simulink model "PID_Block"  (R2020b)
settings: Solver=VariableStepAuto  StartTime=0.0  StopTime=10.0  RelTol=1e-3
values from neighbouring files (symbols this model uses):
  Kd = 300    [mass_damper_pid.m]    (also in mass_damper_pid_improved.m = 0)
  Ki = 50    [mass_damper_pid.m]    (also in mass_damper_pid_improved.m = 0)
  Kp = 500    [mass_damper_pid.m]    (also in mass_damper_pid_improved.m)
settings Model: Creator=Raihan mahmud  LastModifiedBy=Raihan mahmud

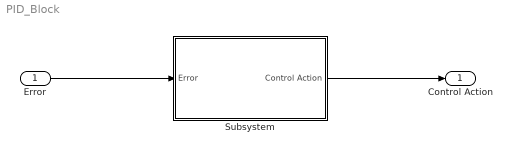
== system PID_Block ==
  Error : Inport
  Subsystem : Subsystem
  Control Action : Outport
  wires:
  Error/1 -> Subsystem/1(Error)
  Subsystem/1(Control Action) -> Control Action/1

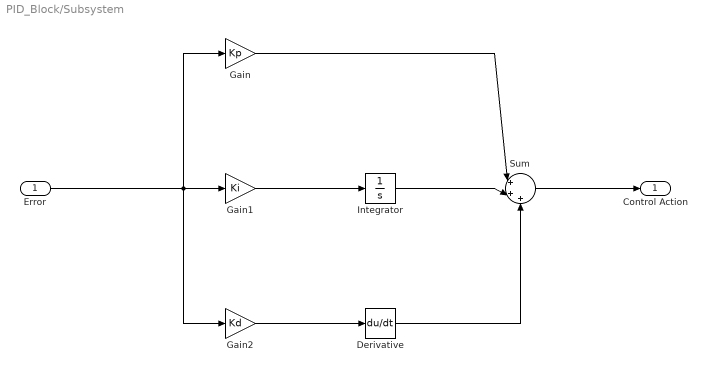
== system PID_Block/Subsystem ==
  Error : Inport
  Derivative : Derivative
  Gain : Gain  Gain=Kp
  Gain1 : Gain  Gain=Ki
  Gain2 : Gain  Gain=Kd
  Integrator : Integrator
  Sum : Sum  Inputs=|+++
  Control Action : Outport
  wires:
  Integrator/1 -> Sum/2
  Error/1 -> Gain2/1, Gain/1, Gain1/1
  Gain2/1 -> Derivative/1
  Sum/1 -> Control Action/1
  Derivative/1 -> Sum/3
  Gain1/1 -> Integrator/1
  Gain/1 -> Sum/1
